simulink model "backward_plant_withoutFeedback"  (R2015a)
settings: Solver=FixedStepDiscrete  StartTime=0.0  StopTime=0.05  RelTol=1e-3
StartFcn:
  | startEventListener
libraries: simulink x1
settings Model: Creator=23933  LastModifiedBy=23933
settings OptimizationCC: BlockReduction=off

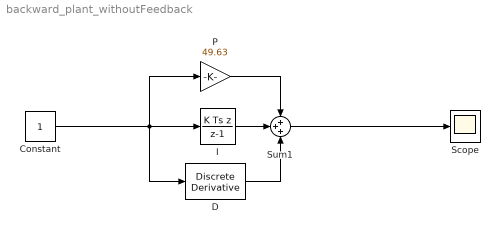
== system backward_plant_withoutFeedback ==
  Constant : Constant
  D : simulink/Discrete/Discrete Derivative  gainval=5.178  ICPrevScaledInput=0.0  OutMin=[]  OutMax=[]  OutDataType=fixdt(1, 16)  OutScaling=2^-10  DoSatur=off
      link override Diff: OutMin=OutMin
  I : DiscreteIntegrator  IntegratorMethod=Integration: Backward Euler  gainval=118.9  InitialConditionSetting=State (most efficient)  SampleTime=0.05
  P : Gain  Gain=49.63
  Scope : Scope
      settings: YMin=-0.12627  YMax=1.13646
  Sum1 : Sum  Inputs=3
  wires:
  Sum1/1 -> Scope/1
  Constant/1 -> I/1, D/1, P/1
  P/1 -> Sum1/1
  D/1 -> Sum1/3
  I/1 -> Sum1/2
